simulink model "rectifiergjr"  (R2024a)
settings: Solver=VariableStepAuto  StartTime=0.0  StopTime=10  RelTol=1e-3  EnableMultiTasking=on
libraries: spsCurrentMeasurementLib x4, spsThyristorLib x4, spsVoltageMeasurementLib x2, spsSeriesRLCBranchLib x1, spsACVoltageSourceLib x1, sps_lib x1
settings Model: Creator=GADDALA JAYARAJU  LastModifiedBy=DELL
settings SolverCC: AlgebraicLoopSolver=TrustRegion
settings DataIOCC: ReturnWorkspaceOutputs=off
settings OptimizationCC: LifeSpan=inf
settings DebuggingCC: UnconnectedInputMsg=warning  UnconnectedOutputMsg=warning  UnconnectedLineMsg=warning  SFUnexpectedBacktrackingDiag=warning  SFNoUnconditionalDefaultTransitionDiag=warning  ArithmeticOperatorsInVariantConditions=warning
settings ModelReferenceCC: EnableRefExpFcnMdlSchedulingChecks=on
settings SFSimCC: SimUseLocalCustomCode=off  CustomCodeUndefinedFunction=UseInterfaceOnly
settings RTWCC: RTWUseLocalCustomCode=off  GPUComputeCapability=3.5
settings CodeAppCC: StateflowObjectComments=on
settings GRTTargetCC: TargetLangStandard=C89/C90 (ANSI)
settings ConfigComp: CovMetricSettings=dw  CovSaveCumulativeToWorkspaceVar=on  CovSaveSingleToWorkspaceVar=on  CovExternalEMLEnable=off
settings SimscapeCC: SimscapeNormalizeSystem=off

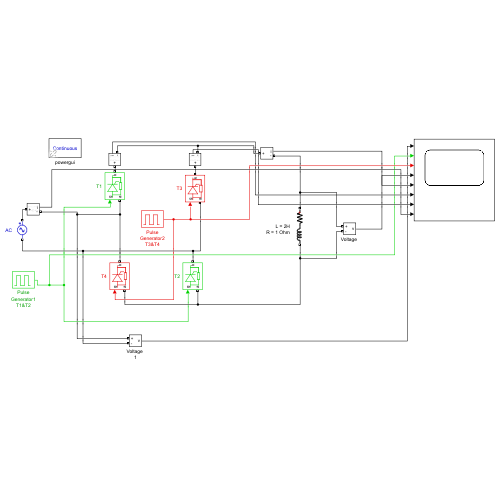
[thumbnail: Simulink's stored preview of the top-level diagram]
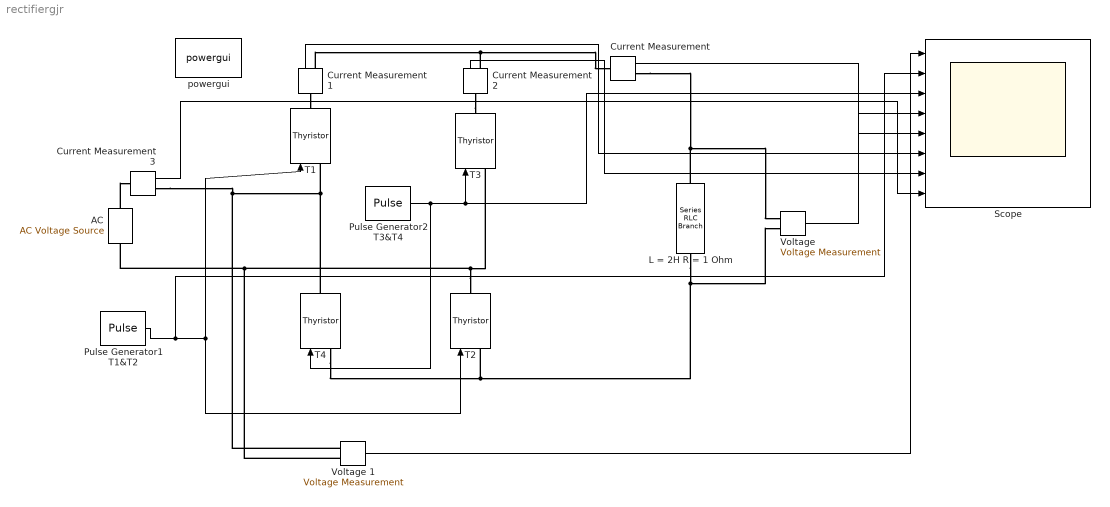
== system rectifiergjr ==
  " L = 2H R = 1 Ohm " : spsSeriesRLCBranchLib/Series RLC Branch  LConnTagsString=__new0  RConnTagsString=__new0  BranchType=RL  Resistance=1  Inductance=2  SetiL0=off  InitialCurrent=0  Capacitance=1e-6  Setx0=off  InitialVoltage=0  Measurements=None
  "AC " : spsACVoltageSourceLib/AC Voltage Source  Amplitude=230  Phase=0  Frequency=50  SampleTime=0  Measurements=None  BusType=swing  Pref=10e3  Qref=0  Qmin=-inf  Qmax=+inf
  Current Measurement{,1..3} (4 alike) : spsCurrentMeasurementLib/Current Measurement  PhasorSimulation=off  OutputType=Complex  PSBequivalent=0
  Pulse Generator1 T1&T2 : DiscretePulseGenerator  PulseType=Time based  Period=0.02  PulseWidth=50  PhaseDelay=0.02*(47/360)
  Pulse Generator2 T3&T4 : DiscretePulseGenerator  PulseType=Time based  Period=0.02  PulseWidth=50  PhaseDelay=0.02*(227/360)
  Scope : Scope  NumInputPorts=8
  T{1..4} (4 alike) : spsThyristorLib/Thyristor  Ron=.00000001  Lon=0  Vf=0  IC=0  Rs=500  Cs=250e-9  Measurements=off
  "Voltage " : spsVoltageMeasurementLib/Voltage Measurement  PhasorSimulation=off  OutputType=Complex  PSBequivalent=0
  Voltage 1 : spsVoltageMeasurementLib/Voltage Measurement  PhasorSimulation=off  OutputType=Complex  PSBequivalent=0
  powergui : sps_lib/powergui  Priority=1  SimulationMode=Continuous  SampleTime=50e-6  frequency=60  Iterations=50  frequencyindice=50  Pbase=100e6  ErrMax=1e-4  UnitsV=kV  UnitsW=MW  buscounter=0  FunctionMessages=off  echomessages=off  EnableUseOfTLC=off  CurrentSourceSwitches=off  DisableSnubberDevices=off  DisableRonSwitches=off  DisableVfSwitches=off  DisplayEquations=off  AutomaticDiscreteSolvers=off  SolverType=Tustin/Backward Euler (TBE)  Interpol=off  ExternalGateDelay=off  methode=off  Ts=10  x0status=blocks  SPID=off  SwTol=0  HookPort=off  NonlinearTolerance=1e-4  nMaxIteration=100  ContinueOnMaxIteration=off  RestoreLinks=warning  ResistiveCurrentMeasurement=off  Frange=[0:2:500]  Ylog=off  Xlog=on  ShowGrid=off  save=off  variable=ZData  structure=0  ZoomFFT=off  StartTime=0.0  cycles=1  DisplayStyle=1  fundamental=60  FreqAxis=off  MaxFrequency=1000  frequencyindicesteady=1  RmsSteady=1  display=off
  wires:
  Pulse Generator1 T1&T2/1 -> Scope/2, T2/1, T1/1
  Pulse Generator2 T3&T4/1 -> T4/1, Scope/3, T3/1
  "Voltage "/1 -> Scope/4
  Current Measurement/1 -> Scope/5
  Voltage 1/1 -> Scope/1
  Current Measurement1/1 -> Scope/6
  Current Measurement2/1 -> Scope/7
  Current Measurement3/1 -> Scope/8
  connections:
  T4/RConn1 -- Voltage 1/LConn1 -- Current Measurement3/RConn1 -- T1/LConn1
  Current Measurement1/RConn1 -- Current Measurement/LConn1 -- Current Measurement2/RConn1
  T2/RConn1 -- Voltage 1/LConn2 -- "AC "/LConn1 -- T3/LConn1
  T4/LConn1 -- " L = 2H R = 1 Ohm "/RConn1 -- "Voltage "/LConn2 -- T2/LConn1
  "Voltage "/LConn1 -- " L = 2H R = 1 Ohm "/LConn1 -- Current Measurement/RConn1
  Current Measurement1/LConn1 -- T1/RConn1
  Current Measurement2/LConn1 -- T3/RConn1
  "AC "/RConn1 -- Current Measurement3/LConn1
